simulink model "simulink_model"  (R2020b)
settings: Solver=ode4  StartTime=0.0  StopTime=T  FixedStep=Ts  RelTol=1e-3
values from neighbouring files (symbols this model uses):
  dq0_1 = dq0(1)    [init.m]
  dq0_2 = dq0(2)    [init.m]
  dq0_3 = dq0(3)    [init.m]
  q0_1 = q0(1)    [init.m]
  q0_2 = q0(2)    [init.m]
  q0_3 = q0(3)    [init.m]
settings Model: Creator=franc  LastModifiedBy=Dell
settings DebuggingCC: SignalInfNanChecking=error

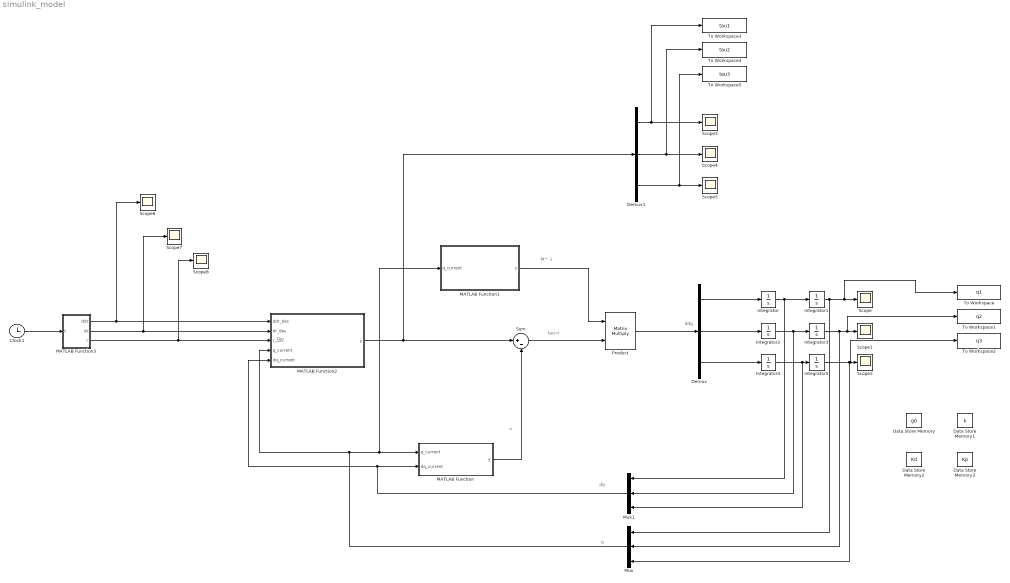
== system simulink_model ==
  note: tau
  note: M^-1
  note: n
  note: q
  note: dq
  note: ddq
  note: tau-n
  Clock1 : Clock
  Data Store Memory : DataStoreMemory  DataStoreName=g0  ReadBeforeWriteMsg=warning  WriteAfterWriteMsg=warning  WriteAfterReadMsg=warning  ShowAdditionalParam=off
  Data Store Memory1 : DataStoreMemory  DataStoreName=k  ReadBeforeWriteMsg=warning  WriteAfterWriteMsg=warning  WriteAfterReadMsg=warning  ShowAdditionalParam=off
  Data Store Memory2 : DataStoreMemory  DataStoreName=Kd  ReadBeforeWriteMsg=warning  WriteAfterWriteMsg=warning  WriteAfterReadMsg=warning  ShowAdditionalParam=off
  Data Store Memory3 : DataStoreMemory  DataStoreName=Kp  ReadBeforeWriteMsg=warning  WriteAfterWriteMsg=warning  WriteAfterReadMsg=warning  ShowAdditionalParam=off
  Demux : Demux  Outputs=3
  Demux1 : Demux  Outputs=3
  Integrator : Integrator  InitialCondition=dq0_1
  Integrator1 : Integrator  InitialCondition=q0_1
  Integrator2 : Integrator  InitialCondition=dq0_2
  Integrator3 : Integrator  InitialCondition=q0_2
  Integrator4 : Integrator  InitialCondition=dq0_3
  Integrator5 : Integrator  InitialCondition=q0_3
  MATLAB Function : MATLAB Function  TreatAsAtomicUnit=on
  MATLAB Function1 : MATLAB Function  TreatAsAtomicUnit=on
  MATLAB Function2 : MATLAB Function  TreatAsAtomicUnit=on
  MATLAB Function3 : MATLAB Function  TreatAsAtomicUnit=on
  Mux : Mux  Inputs=3
  Mux1 : Mux  Inputs=3
  Product : Product  Multiplication=Matrix(*)
  Scope{,1..8} (9 alike) : Scope
  Sum : Sum  Inputs=|+-
  To Workspace : ToWorkspace  VariableName=q1  SaveFormat=Structure With Time  SampleTime=-1
  To Workspace1 : ToWorkspace  VariableName=q2  SaveFormat=Structure With Time  SampleTime=-1
  To Workspace2 : ToWorkspace  VariableName=q3  SaveFormat=Structure With Time  SampleTime=-1
  To Workspace3 : ToWorkspace  VariableName=tau1  SaveFormat=Structure With Time  SampleTime=-1
  To Workspace4 : ToWorkspace  VariableName=tau2  SaveFormat=Structure With Time  SampleTime=-1
  To Workspace5 : ToWorkspace  VariableName=tau3  SaveFormat=Structure With Time  SampleTime=-1
  wires:
  Integrator/1 -> Mux1/1, Integrator1/1
  Integrator2/1 -> Mux1/2, Integrator3/1
  Integrator4/1 -> Mux1/3, Integrator5/1
  Integrator1/1 -> Mux/1, To Workspace/1, Scope/1
  Integrator3/1 -> To Workspace1/1, Scope1/1, Mux/2
  Integrator5/1 -> Mux/3, To Workspace2/1, Scope2/1
  Demux/1 -> Integrator/1
  Demux/2 -> Integrator2/1
  Demux/3 -> Integrator4/1
  MATLAB Function2/1(y) -> Demux1/1, Sum/1
  Sum/1 -> Product/2
  Product/1 -> Demux/1
  MATLAB Function/1(y) -> Sum/2
  Mux1/1 -> MATLAB Function2/5(dq_current), MATLAB Function/2(dq_current)
  Mux/1 -> MATLAB Function2/4(q_current), MATLAB Function1/1(q_current), MATLAB Function/1(q_current)
  MATLAB Function1/1(y) -> Product/1
  MATLAB Function3/1(ddr) -> Scope6/1, MATLAB Function2/1(ddr_des)
  MATLAB Function3/2(dr) -> Scope7/1, MATLAB Function2/2(dr_des)
  MATLAB Function3/3(r) -> Scope8/1, MATLAB Function2/3(r_des)
  Demux1/3 -> To Workspace5/1, Scope5/1
  Demux1/2 -> To Workspace4/1, Scope4/1
  Demux1/1 -> To Workspace3/1, Scope3/1
  Clock1/1 -> MATLAB Function3/1(t)

== matlab function simulink_model/MATLAB Function ==
  settings: updateMethod=DISCRETE
  data: q_current input; y output; dq_current input
function y = evaluate_n(q_current, dq_current)

q1 = q_current(1);
q2 = q_current(2);
q3 = q_current(3);
dq1 = dq_current(1);
dq2 = dq_current(2);
dq3 = dq_current(3);

% global g0;
L = 1;
dc1 = 1/2 * L;
dc2 = 1/2 * L;
dc3 = 1/2 * L;
m1 = 10;
m2 = 10;
m3 = 10;
I1 = 1/12 * m1 * L^2;
I2 = 1/12 * m2 * L^2;
I3 = 1/12 * m3 * L^2;
g0=0;

n=zeros(3,1);
n(1)=g0*m3*(L*cos(q1 + q2) + L*cos(q1) + dc3*cos(q1 + q2 + q3)) - L*(dc3*dq2^2*m3*sin(q2 + q3) + dc3*dq3^2*m3*sin(q2 + q3) + L*dq2^2*m3*sin(q2) + dc2*dq2^2*m2*sin(q2) + dc3*dq3^2*m3*sin(q3) + 2*dc3*dq1*dq2*m3*sin(q2 + q3) + 2*dc3*dq1*dq3*m3*sin(q2 + q3) + 2*dc3*dq2*dq3*m3*sin(q2 + q3) + 2*L*dq1*dq2*m3*sin(q2) + 2*dc2*dq1*dq2*m2*sin(q2) + 2*dc3*dq1*dq3*m3*sin(q3) + 2*dc3*dq2*dq3*m3*sin(q3)) + g0*m2*(dc2*cos(q1 + q2) + L*cos(q1)) + dc1*g0*m1*cos(q1);
n(2)=L*(dc3*dq1^2*m3*sin(q2 + q3) + L*dq1^2*m3*sin(q2) + dc2*dq1^2*m2*sin(q2) - dc3*dq3^2*m3*sin(q3) - 2*dc3*dq1*dq3*m3*sin(q3) - 2*dc3*dq2*dq3*m3*sin(q3)) + g0*m3*(L*cos(q1 + q2) + dc3*cos(q1 + q2 + q3)) + dc2*g0*m2*cos(q1 + q2);
n(3)=dc3*g0*m3*cos(q1 + q2 + q3) + L*dc3*m3*(dq1^2*sin(q3) + dq2^2*sin(q3) + dq1^2*sin(q2 + q3) + 2*dq1*dq2*sin(q3));
y=n;

== matlab function simulink_model/MATLAB Function3 ==
  data: t input; ddr output size=2; dr output size=2; r output size=2
function [ddr, dr, r] = evaluate_trajectory(t)

T=5;

%% LINEAR TRAJECTORY
% 
% tau_t = t/T;
% s = -2*tau_t^3 + 3*tau_t^2;
% ds = (6*t)/T^2 - (6*t^2)/T^3;
% dds = 6/T^2 - (12*t)/T^3;
% start = [1.3660; 2.3660];
% finish = [2.5; 0];
% r = start + s*(finish-start);
% dr = (finish-start)*ds;
% ddr = (finish-start)*dds;

%% CIRCULAR TRAJECTORY

h = 0;
if t > T
    h = 1
end
tau_t = t/T - h;
center = [1.5; 1];
radius = 0.5;
s = -2*tau_t^3 + 3*tau_t^2;
ds = (6*t)/T^2 - (6*t^2)/T^3;
dds = 6/T^2 - (12*t)/T^3;
r = center + radius * [cos(s* 2*pi) ; sin(s * 2 * pi)];
dr = 2*pi * radius * [-sin(s*2*pi); cos(2*s*pi)] * ds;
ddr = (2 *pi)^2 * radius * [-cos(s*2*pi); -sin(2*s*pi)]* dds;

%% STAY AT THE POINT
% start = [1.3660; 2.3660];
% r = start;
% dr = [0; 0];
% ddr = [0; 0];

== matlab function simulink_model/MATLAB Function1 ==
  data: q_current input size=3; y output
function y = evaluate_inv_M(q_current)

q1 = q_current(1);
q2 = q_current(2);
q3 = q_current(3);

L = 1;
dc1 = 1/2 * L;
dc2 = 1/2 * L;
dc3 = 1/2 * L;
m1 = 10;
m2 = 10;
m3 = 10;
I1 = 1/12 * m1 * L^2;
I2 = 1/12 * m2 * L^2;
I3 = 1/12 * m3 * L^2;

M=zeros(3,3);
M(1,1)=I1 + I2 + I3 + L^2*m2 + 2*L^2*m3 + 2*cos(q2)*(m3*L^2 + dc2*m2*L) + dc1^2*m1 + dc2^2*m2 + dc3^2*m3 + 2*L*dc3*m3*cos(q2 + q3) + 2*L*dc3*m3*cos(q3);
M(1,2)=I2 + I3 + L^2*m3 + cos(q2)*(m3*L^2 + dc2*m2*L) + dc2^2*m2 + dc3^2*m3 + L*dc3*m3*cos(q2 + q3) + 2*L*dc3*m3*cos(q3);
M(1,3)=I3 + dc3^2*m3 + L*dc3*m3*cos(q2 + q3) + L*dc3*m3*cos(q3);
M(2,2)=m3*L^2 + 2*m3*cos(q3)*L*dc3 + m2*dc2^2 + m3*dc3^2 + I2 + I3;
M(2,3)=m3*dc3^2 + L*m3*cos(q3)*dc3 + I3;
M(3,3)=m3*dc3^2 + I3;
M(2,1)=M(1,2);
M(3,1)=M(1,3);
M(3,2)=M(2,3);

M_inv=inv(M);

y = M_inv;

== matlab function simulink_model/MATLAB Function2 ==
  settings: updateMethod=DISCRETE
  data: ddr_des input; dr_des input; r_des input; q_current input size=3; y output size=3; dq_current input size=3
function y = compute_tau(ddr_des, dr_des, r_des, q_current, dq_current)


g0 = 0;
Kp = diag([400,400]);
Kd = diag([40,40]);
k = 2;


q1 = q_current(1);
q2 = q_current(2);
q3 = q_current(3);

dq1 = dq_current(1);
dq2 = dq_current(2);
dq3 = dq_current(3);
dq=[dq1;dq2;dq3];

M=zeros(3,3);
M(1,1)=10*cos(q2 + q3) + 30*cos(q2) + 10*cos(q3) + 40;
M(1,2)=5*cos(q2 + q3) + 15*cos(q2) + 10*cos(q3) + 50/3;
M(1,3)=5*cos(q2 + q3) + 5*cos(q3) + 10/3;
M(2,2)=10*cos(q3) + 50/3;
M(2,3)=5*cos(q3) + 10/3;
M(3,3)=10/3;
M(2,1)=M(1,2);
M(3,1)=M(1,3);
M(3,2)=M(2,3);

n=zeros(3,1);
n(1)=5*g0*(cos(q1 + q2 + q3) + 3*cos(q1 + q2) + 5*cos(q1)) - 5*dq3^2*sin(q3) - 15*dq2^2*sin(q2) - 5*dq2^2*sin(q2 + q3) - 5*dq3^2*sin(q2 + q3) - 30*dq1*dq2*sin(q2) - 10*dq1*dq3*sin(q3) - 10*dq2*dq3*sin(q3) - 10*dq1*dq2*sin(q2 + q3) - 10*dq1*dq3*sin(q2 + q3) - 10*dq2*dq3*sin(q2 + q3);
n(2)=15*dq1^2*sin(q2) - 5*dq3^2*sin(q3) + 5*g0*(cos(q1 + q2 + q3) + 3*cos(q1 + q2)) + 5*dq1^2*sin(q2 + q3) - 10*dq1*dq3*sin(q3) - 10*dq2*dq3*sin(q3);
n(3)=5*dq1^2*sin(q3) + 5*dq2^2*sin(q3) + 5*dq1^2*sin(q2 + q3) + 5*g0*cos(q1 + q2 + q3) + 10*dq1*dq2*sin(q3);

J=zeros(2,3);
J(1,:) = [- sin(q1 + q2 + q3) - sin(q1 + q2) - sin(q1), - sin(q1 + q2 + q3) - sin(q1 + q2), -sin(q1 + q2 + q3)];
J(2,:) = [cos(q1 + q2 + q3) + cos(q1 + q2) + cos(q1),   cos(q1 + q2 + q3) + cos(q1 + q2),  cos(q1 + q2 + q3)];
dJ=zeros(2,3);
dJ(1,:)= [- 3*cos(q1 + q2 + q3) - 2*cos(q1 + q2) - cos(q1), - 3*cos(q1 + q2 + q3) - 2*cos(q1 + q2), -3*cos(q1 + q2 + q3)];
dJ(2,:)= [- 3*sin(q1 + q2 + q3) - 2*sin(q1 + q2) - sin(q1), - 3*sin(q1 + q2 + q3) - 2*sin(q1 + q2), -3*sin(q1 + q2 + q3)];

M_inv = M^-1;
M_weighted = M^(k-2);

r = [cos(q1) + cos(q1+q2) + cos(q1+q2+q3); sin(q1) + sin(q1+q2) + sin(q1+q2+q3)];
dr = J*dq;

ddr = ddr_des + Kd*(dr_des - dr) + Kp*(r_des - r);

%% Without damping factor
% tau0 = [0;0;0];
%% With damping factor
tau0 = -M*[Kd [0 0]'; 0 0 Kd(1,1)]*dq;

J_pseudo_weighted = M_weighted * (J' * pinv(J * M_weighted * J'));
tau = M * (J_pseudo_weighted * (ddr - dJ * dq + J * M_inv * n)) + M * ((eye(3) - J_pseudo_weighted * J) * (M_inv * tau0));

y = tau;
